simulink model "LAB6T2"  (R2018b)
settings: Solver=ode45  StartTime=0.0  StopTime=3600  RelTol=1e-1
libraries: aerolibanim x1
settings Model: Creator=aloisia  LastModifiedBy=aloisia

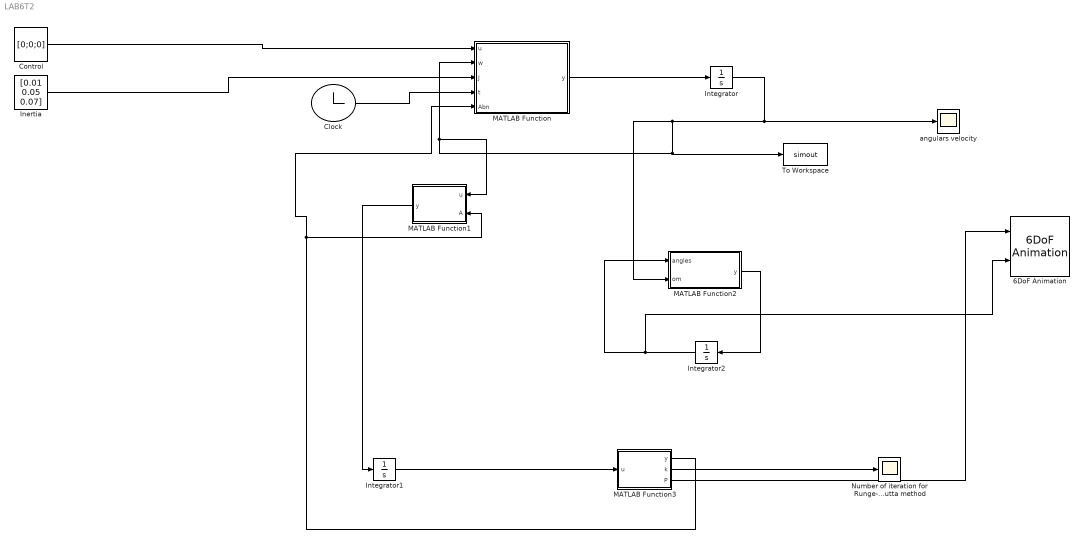
== system LAB6T2 ==
  6DoF Animation : aerolibanim/6DoF Animation  u1=[0 4000 -2000 2000 -5000 -3000]  u2=0.07  u3=800  u4=[4000 0 -5000]  u5=Fixed position  u6=[2000 500 -3150]  u7=10  u8=on
      settings: SourceProductName=Aerospace Blockset
  Clock : Clock
  "Control " : Constant  Tag=J  Description=J  Value=[0;0;0]
  "Inertia " : Constant  Tag=J  Description=J  Value=[0.01 0.05 0.07]
  Integrator : Integrator  InitialCondition=[0.01;0.01;7.2911e-1]
  Integrator1 : Integrator  InitialCondition=eye(3)
  Integrator2 : Integrator  InitialCondition=[0;0;0]
  MATLAB Function : MATLAB Function  TreatAsAtomicUnit=on
  MATLAB Function1 : MATLAB Function  TreatAsAtomicUnit=on
  MATLAB Function2 : MATLAB Function  TreatAsAtomicUnit=on
  MATLAB Function3 : MATLAB Function  TreatAsAtomicUnit=on
  Number of iteration for Runge-Kutta method : Scope
  To Workspace : ToWorkspace  VariableName=simout  SampleTime=-1
  "angulars velocity " : Scope
  wires:
  Integrator2/1 -> 6DoF Animation/2, MATLAB Function2/1(angles)
  MATLAB Function3/1(y) -> MATLAB Function/5(Abn), MATLAB Function1/2(A)
  MATLAB Function2/1(y) -> Integrator2/1
  Integrator/1 -> MATLAB Function2/2(om), To Workspace/1, MATLAB Function/2(w), MATLAB Function1/1(u), "angulars velocity "/1
  MATLAB Function3/3(P) -> 6DoF Animation/1
  MATLAB Function1/1(y) -> Integrator1/1
  Clock/1 -> MATLAB Function/4(t)
  MATLAB Function/1(y) -> Integrator/1
  MATLAB Function3/2(k) -> Number of iteration for Runge-Kutta method/1
  "Inertia "/1 -> MATLAB Function/3(J)
  Integrator1/1 -> MATLAB Function3/1(u)
  "Control "/1 -> MATLAB Function/1(u)

== matlab function LAB6T2/MATLAB Function1 ==
  data: u input; y output; A input
function y = kinematics(u,A)


W=[0 -u(3) u(2); u(3) 0 -u(1); -u(2) -u(1) 0];

Adot=-W*A ;

y=Adot ;
end

== matlab function LAB6T2/MATLAB Function ==
  data: u input; w input; y output; J input; t input; Abn input
function y  = euler(u,w,J,t,Abn)

%Set Data
Ix=J(1); Iy=J(2); Iz=J(3) ;
wx=w(1) ; wy=w(2); wz=w(3);
wdot=[0;0;0];
%%Gravity Gradiant
 R=42168;
 n=(398600/(R^3))^0.5 ;
Aln=[cos(n*t+0.1) sin(n*t+0.1) 0 ; -sin(n*t+0.1) cos(n*t+0.1) 0; 0 0 1];

Abl=Abn*(Aln');
c=Abl*[1;0;0];
Ma1=(3*(n^2))*((Iz-Iy)*c(3)*c(2));
Ma2=(3*(n^2))*((Ix-Iz)*c(1)*c(3));
Ma3=(3*(n^2))*((Iy-Ix)*c(1)*c(2));

%% Euler Equation
wdot(1)= ((Iy-Iz)/Ix)*wy*wz+u(1)/Ix+Ma1/Ix;
wdot(2)= ((Iz-Ix)/Iy)*wx*wz+u(2)/Iy+Ma2/Iy;
wdot(3)= ((Ix-Iy)/Iz)*wx*wy+u(3)/Iz+Ma3/Iz;


y = wdot;
Aln = Aln;
end

== matlab function LAB6T2/MATLAB Function2 ==
  data: angles input; y output; om input
function y = fcn(angles,om)

% This function provides the calculation of A by using 
% Phi, theta, psi and omega.Radiants
phi = angles(1);
theta = angles(2);
psi = angles(3);

phidot = (om(1)*cos(psi) - om(2)*sin(psi)) / cos(theta);
thetadot = om(2)*cos(psi) + om(1)*sin(psi);
psidot = om(3) - (om(1)*cos(psi) - om(2)*sin(psi))* sin(theta)/cos(theta);
anglesdot = [phidot; thetadot; psidot];

y = anglesdot;
end

== matlab function LAB6T2/MATLAB Function3 ==
  data: u input; y output; k output; P output
function [y,k,P]  = ortho(u)

c=1; A=u; k=0;
while c>0.000001

A=(1.5.*A)-(A*(A')*A./2) ; % Runge-Kutta method
c=trace((eye(3)-(A')*A)) ; % error
k=k+1 ; %counter
end

z=k;
y=A ;
P = A * [1;0;0];

end
